simulink model "parallelizationTest"  (R2017a)
settings: Solver=FixedStepAuto  StartTime=0.0  StopTime=10  FixedStep=0.1  RelTol=1e-3
settings Model: Creator=TSu  LastModifiedBy=TSu
settings SolverCC: AutoInsertRateTranBlk=on
settings DebuggingCC: RootOutportRequireBusObject=error  StrictBusMsg=ErrorOnBusTreatedAsVector
settings HardwareCC: ProdBitPerLong=64  ProdBitPerPointer=32  ProdBitPerSizeT=32  ProdBitPerPtrDiffT=32  ProdLargestAtomicFloat=None  ProdHWDeviceType=Generic->Custom
settings SFSimCC: SimCustomHeaderCode="#include \"time_par_tests.h\""  SimUserSources=time_par_tests.c
settings RTWCC: SystemTargetFile=NIVeriStand_Linux_64.tlc  GenCodeOnly=on  PackageGeneratedCodeAndArtifacts=on  PackageName=testParallelization  TemplateMakefile=NIVeriStand_Linux_64.tmf  Description=NI Linux Real-Time (64-bit) Target
settings STFCustomTargetCC: TargetLangStandard=C99 (ISO)  MatFileLogging=on  MATLABClassNameForMDSCustomization=Simulink.SoftwareTarget.TargetSpecificTriggerConfigurationBase  SystemTargetFile=NIVeriStand_Linux_64.tlc

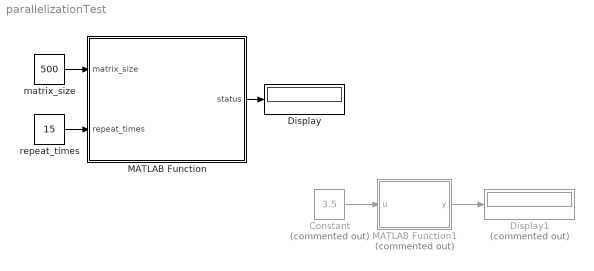
== system parallelizationTest ==
  Constant : Constant  Commented=on  Value=3.5
  Display : Display
      settings: Decimation=2
  Display1 : Display  Commented=on
  MATLAB Function : MATLAB Function  TreatAsAtomicUnit=on
  MATLAB Function1 : MATLAB Function  Commented=on  TreatAsAtomicUnit=on
  matrix_size : Constant  Value=500
  repeat_times : Constant  Value=15
  wires:
  matrix_size/1 -> MATLAB Function/1(matrix_size)
  repeat_times/1 -> MATLAB Function/2(repeat_times)
  MATLAB Function/1(status) -> Display/1
  Constant/1 -> MATLAB Function1/1(u)
  MATLAB Function1/1(y) -> Display1/1

== matlab function parallelizationTest/MATLAB Function1 ==
  data: u input; y output
function y = callingDoubleIt(u)
y = 0.0;
y = coder.ceval('doubleIt',u);

== matlab function parallelizationTest/MATLAB Function ==
  data: matrix_size input; status output; repeat_times input
function status = time_par_tests(matrix_size, repeat_times)
% time_par_tests: Perform a parallization test (baseline)

status = 0;
status = coder.ceval('time_par_tests',matrix_size, repeat_times);

end
